simulink model "Normal_Calc"  (R2017b)
settings: Solver=FixedStepDiscrete  StartTime=0.0  StopTime=10.0  RelTol=1e-3
settings Model: Creator=engdo  LastModifiedBy=engdo
settings OptimizationCC: DefaultParameterBehavior=Inlined  PassReuseOutputArgsAs=Individual arguments
settings DebuggingCC: ParameterTunabilityLossMsg=error
settings SFSimCC: MATLABDynamicMemAlloc=off
settings RTWCC: SystemTargetFile=ert.tlc  GenCodeOnly=on  TemplateMakefile=ert_default_tmf  GenerateReport=on  IncludeHyperlinkInReport=on  LaunchReport=on  GenerateTraceInfo=on  GenerateTraceReport=on  GenerateTraceReportSl=on  GenerateTraceReportSf=on  GenerateTraceReportEml=on  GenerateWebview=on
settings CodeAppCC: ForceParamTrailComments=on  IgnoreCustomStorageClasses=off  OperatorAnnotations=on  SimulinkDataObjDesc=on  SFDataObjDesc=on  InsertBlockDesc=on
settings ERTTargetCC: TargetLangStandard=C99 (ISO)  GenerateSampleERTMain=on  InlinedParameterPlacement=NonHierarchical  ERTCustomFileTemplate=example_file_process.tlc  EnableUserReplacementTypes=on

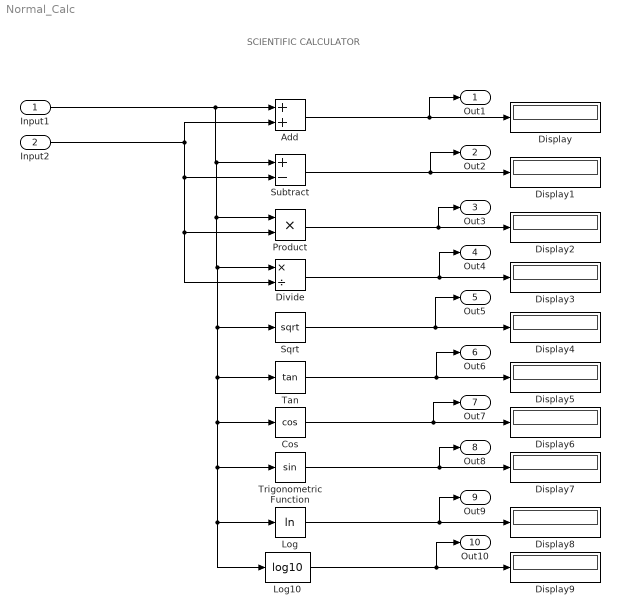
== system Normal_Calc ==
  note: SCIENTIFIC CALCULATOR
  Input1 : Inport  OutDataTypeStr=double
  Input2 : Inport  Port=2  OutDataTypeStr=double
  Add : Sum
  Cos : Trigonometry  Operator=cos
  Display{,1..9} (10 alike) : Display
  Divide : Product  Inputs=*/
  Log : Math  Operator=log  SaturateOnIntegerOverflow=on
  Log10 : Math  Operator=log10  RndMeth=Zero  SaturateOnIntegerOverflow=on
  Product : Product
  Sqrt : Sqrt  SaturateOnIntegerOverflow=on
  Subtract : Sum  Inputs=+-
  Tan : Trigonometry  Operator=tan
  Trigonometric Function : Trigonometry
  Out1 : Outport  OutDataTypeStr=double
  Out2 : Outport  Port=2  OutDataTypeStr=double
  Out3 : Outport  Port=3  OutDataTypeStr=double
  Out4 : Outport  Port=4  OutDataTypeStr=double
  Out5 : Outport  Port=5  OutDataTypeStr=double
  Out6 : Outport  Port=6  OutDataTypeStr=double
  Out7 : Outport  Port=7  OutDataTypeStr=double
  Out8 : Outport  Port=8  OutDataTypeStr=double
  Out9 : Outport  Port=9  OutDataTypeStr=double
  Out10 : Outport  Port=10  OutDataTypeStr=double
  wires:
  Add/1 -> Out1/1, Display/1
  Subtract/1 -> Out2/1, Display1/1
  Product/1 -> Out3/1, Display2/1
  Divide/1 -> Out4/1, Display3/1
  Sqrt/1 -> Out5/1, Display4/1
  Tan/1 -> Out6/1, Display5/1
  Cos/1 -> Out7/1, Display6/1
  Trigonometric Function/1 -> Out8/1, Display7/1
  Input1/1 -> Log10/1, Log/1, Trigonometric Function/1, Cos/1, Tan/1, Sqrt/1, Divide/1, Product/1, Subtract/1, Add/1
  Input2/1 -> Add/2, Divide/2, Product/2, Subtract/2
  Log/1 -> Out9/1, Display8/1
  Log10/1 -> Out10/1, Display9/1
